simulink model "wrapper_ASW"  (R2024b)
settings: Solver=FixedStepDiscrete  StartTime=0.0  StopTime=10.0  FixedStep=0.001  MaxStep=0.001  RelTol=1e-3
libraries: simulink x2, CTRL x1, ESTS x1, INP x1, FUSI x1, OUT x1
settings Model: Creator=blatak  LastModifiedBy=blatak
settings ModelReferenceCC: EnableRefExpFcnMdlSchedulingChecks=on
settings RTWCC: GPUComputeCapability=3.5

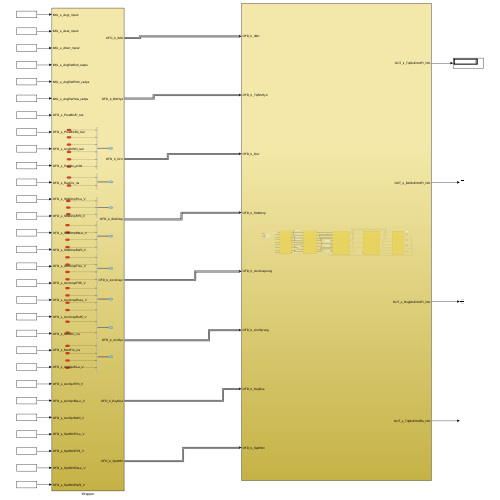
[thumbnail: Simulink's stored preview of the top-level diagram]
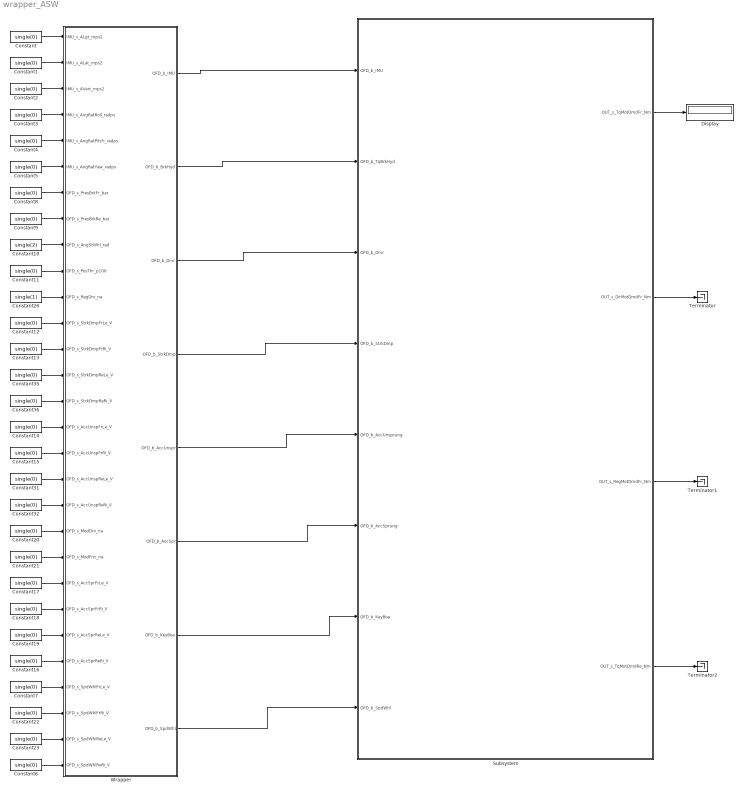
== system wrapper_ASW ==
  Constant{,1..9,11..23,31..32,35..36} (27 alike) : Constant  Value=single(0)
  Constant10 : Constant  Value=single(2)
  Constant26 : Constant  Value=single(1)
  Display : Display
  Subsystem : Subsystem
  Terminator : Terminator
  Terminator1 : Terminator
  Terminator2 : Terminator
  Wrapper : Subsystem
  wires:
  Wrapper/1(OFD_b_IMU) -> Subsystem/1(OFD_b_IMU)
  Wrapper/2(OFD_b_BrkHyd) -> Subsystem/2(OFD_b_TqBrkHyd)
  Wrapper/3(OFD_b_Drvr) -> Subsystem/3(OFD_b_Drvr)
  Wrapper/7(OFD_b_KeyBoa) -> Subsystem/7(OFD_b_KeyBoa)
  Constant/1 -> Wrapper/1(IMU_s_ALgt_mps2)
  Constant1/1 -> Wrapper/2(IMU_s_ALat_mps2)
  Constant2/1 -> Wrapper/3(IMU_s_AVert_mps2)
  Constant3/1 -> Wrapper/4(IMU_s_AngRatRoll_radps)
  Constant4/1 -> Wrapper/5(IMU_s_AngRatPitch_radps)
  Constant5/1 -> Wrapper/6(IMU_s_AngRatYaw_radps)
  Constant8/1 -> Wrapper/7(OFD_s_PresBrkFr_bar)
  Constant9/1 -> Wrapper/8(OFD_s_PresBrkRe_bar)
  Constant10/1 -> Wrapper/9(OFD_s_AngStWhl_rad)
  Constant11/1 -> Wrapper/10(OFD_s_PosThr_p100)
  Constant12/1 -> Wrapper/12(OFD_s_StrkDmpFrLe_V)
  Constant13/1 -> Wrapper/13(OFD_s_StrkDmpFrRi_V)
  Constant14/1 -> Wrapper/16(OFD_s_AccUnspFrLe_V)
  Constant15/1 -> Wrapper/17(OFD_s_AccUnspFrRi_V)
  Constant20/1 -> Wrapper/20(OFD_s_ModDrv_na)
  Constant21/1 -> Wrapper/21(OFD_s_ModFric_na)
  Constant26/1 -> Wrapper/11(OFD_s_RegDrv_na)
  Subsystem/1(OUT_s_TqMotDmdFr_Nm) -> Display/1
  Subsystem/2(OUT_s_DirMotDmdFr_Nm) -> Terminator/1
  Subsystem/3(OUT_s_RegMotDmdFr_Nm) -> Terminator1/1
  Subsystem/4(OUT_s_TqMotDmdRe_Nm) -> Terminator2/1
  Constant31/1 -> Wrapper/18(OFD_s_AccUnspReLe_V)
  Constant32/1 -> Wrapper/19(OFD_s_AccUnspReRi_V)
  Constant35/1 -> Wrapper/14(OFD_s_StrkDmpReLe_V)
  Constant36/1 -> Wrapper/15(OFD_s_StrkDmpReRi_V)
  Constant17/1 -> Wrapper/22(OFD_s_AccSprFrLe_V)
  Constant18/1 -> Wrapper/23(OFD_s_AccSprFrRi_V)
  Constant19/1 -> Wrapper/24(OFD_s_AccSprReLe_V)
  Constant16/1 -> Wrapper/25(OFD_s_AccSprReRi_V)
  Wrapper/6(OFD_b_AccSpr) -> Subsystem/6(OFD_b_AccSprung)
  Wrapper/5(OFD_b_AccUnspr) -> Subsystem/5(OFD_b_AccUnsprung)
  Wrapper/4(OFD_b_StrkDmp) -> Subsystem/4(OFD_b_StrkDmp)
  Constant7/1 -> Wrapper/26(OFD_s_SpdWhlFrLe_V)
  Constant22/1 -> Wrapper/27(OFD_s_SpdWhlFrRi_V)
  Constant23/1 -> Wrapper/28(OFD_s_SpdWhlReLe_V)
  Constant6/1 -> Wrapper/29(OFD_s_SpdWhlReRi_V)
  Wrapper/8(OFD_b_SpdWhl) -> Subsystem/8(OFD_b_SpdWhl)

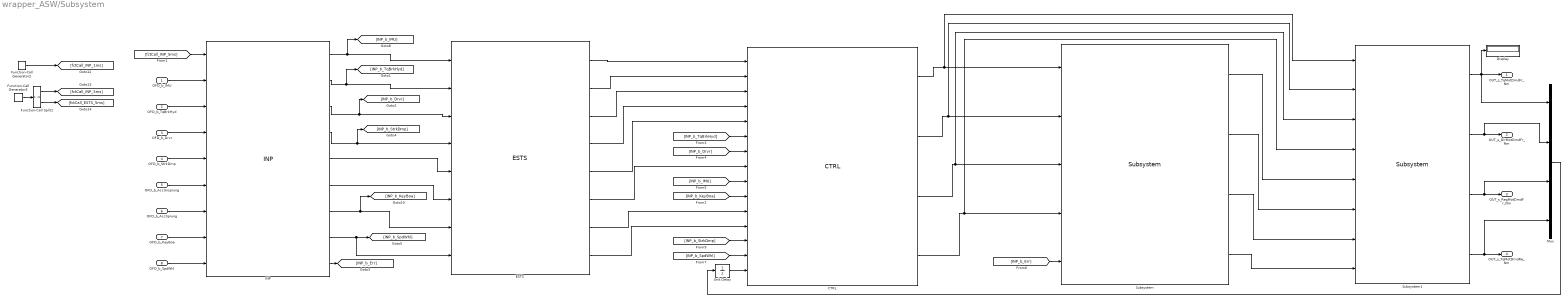
== system wrapper_ASW/Subsystem ==
  OFD_b_IMU : Inport
  OFD_b_TqBrkHyd : Inport  Port=2
  OFD_b_Drvr : Inport  Port=3
  OFD_b_StrkDmp : Inport  Port=4
  OFD_b_AccUnsprung : Inport  Port=5
  OFD_b_AccSprung : Inport  Port=6
  OFD_b_KeyBoa : Inport  Port=7
  OFD_b_SpdWhl : Inport  Port=8
  CTRL : CTRL/CTRL  SystemSampleTime=-1  VariantActivationTime=update diagram  AllowFlexibleInterface=on  Latency=0  AutoFrameSizeCalculation=off
  Display : Display
  ESTS : ESTS/ESTS  SystemSampleTime=-1  VariantActivationTime=update diagram  AllowFlexibleInterface=on  Latency=0  AutoFrameSizeCalculation=off
  Function-Call Generator2 : simulink/Ports & Subsystems/Function-Call Generator  sample_time=1  numberOfIterations=1  DisallowWideOutput=off
  Function-Call Generator3 : simulink/Ports & Subsystems/Function-Call Generator  sample_time=0.005  numberOfIterations=1  DisallowWideOutput=off
  Function-Call Split1 : FunctionCallSplit  IconShape=distinctive  NumOutputPorts=2  OutputPortLayout=default
  INP : INP/INP  SystemSampleTime=-1  VariantActivationTime=update diagram  AllowFlexibleInterface=on  Latency=0  AutoFrameSizeCalculation=off
      link override Function-Call Subsystem1/Bus Selector2: OutputSignals=OFD_s_AngStWhl_rad,OFD_s_PosThr_p100,OFD_s_RegDrv_na
  Mux : Mux
  Subsystem : FUSI/Subsystem  SystemSampleTime=-1  VariantActivationTime=update diagram  AllowFlexibleInterface=on  Latency=0  AutoFrameSizeCalculation=off
  Subsystem1 : OUT/Subsystem  SystemSampleTime=-1  VariantActivationTime=update diagram  AllowFlexibleInterface=on  Latency=0  AutoFrameSizeCalculation=off
  Unit Delay : UnitDelay  SampleTime=-1  HasFrameUpgradeWarning=on
  OUT_s_TqMotDmdFr_Nm : Outport
  OUT_s_DirMotDmdFr_Nm : Outport  Port=2
  OUT_s_RegMotDmdFr_Nm : Outport  Port=3
  OUT_s_TqMotDmdRe_Nm : Outport  Port=4
  wires:
  OFD_b_IMU/1 -> INP/2
  [fctCall_INP_5ms] -> INP/1
  OFD_b_Drvr/1 -> INP/4
  INP/3 -> [INP_b_Drvr], ESTS/3
  Function-Call Generator2/1 -> [fctCall_INP_1ms]
  Function-Call Generator3/1 -> Function-Call Split1/1
  INP/1 -> ESTS/1, [INP_b_IMU]
  Function-Call Split1/1 -> [fctCall_INP_5ms]
  Function-Call Split1/2 -> [fctCall_ESTS_5ms]
  ESTS/7 -> CTRL/11
  [INP_b_KeyBoa] -> CTRL/10
  [INP_b_Drvr] -> CTRL/7
  [INP_b_TqBrkHyd] -> CTRL/6
  ESTS/6 -> CTRL/8
  [INP_b_IMU] -> CTRL/9
  CTRL/1 -> Subsystem1/1, Subsystem/1
  CTRL/2 -> Subsystem1/2, Subsystem/2
  CTRL/3 -> Subsystem1/3, Subsystem/3
  CTRL/4 -> Subsystem1/4, Subsystem/4
  Subsystem1/1 -> Display/1, Mux/1, OUT_s_TqMotDmdFr_Nm/1
  Subsystem1/2 -> Mux/2, OUT_s_DirMotDmdFr_Nm/1
  Subsystem1/3 -> Mux/3, OUT_s_RegMotDmdFr_Nm/1
  Subsystem1/4 -> Mux/4, OUT_s_TqMotDmdRe_Nm/1
  [INP_b_StrkDmp] -> CTRL/13
  OFD_b_TqBrkHyd/1 -> INP/3
  OFD_b_StrkDmp/1 -> INP/5
  OFD_b_AccUnsprung/1 -> INP/6
  OFD_b_AccSprung/1 -> INP/7
  OFD_b_KeyBoa/1 -> INP/8
  INP/2 -> ESTS/2, [INP_b_TqBrkHyd]
  INP/4 -> [INP_b_StrkDmp], ESTS/4
  INP/5 -> ESTS/5
  INP/6 -> ESTS/6
  INP/7 -> ESTS/7, [INP_b_KeyBoa]
  ESTS/1 -> CTRL/1
  ESTS/2 -> CTRL/2
  ESTS/3 -> CTRL/3
  ESTS/4 -> CTRL/4
  ESTS/5 -> CTRL/5
  ESTS/8 -> CTRL/12
  [INP_b_Err] -> Subsystem/5
  Subsystem/1 -> Subsystem1/5
  Subsystem/2 -> Subsystem1/6
  Subsystem/3 -> Subsystem1/7
  Subsystem/4 -> Subsystem1/8
  OFD_b_SpdWhl/1 -> INP/9
  INP/8 -> [INP_b_SpdWhl], ESTS/8
  INP/9 -> [INP_b_Err]
  [INP_b_SpdWhl] -> CTRL/14
  Mux/1 -> Unit Delay/1
  Unit Delay/1 -> CTRL/15

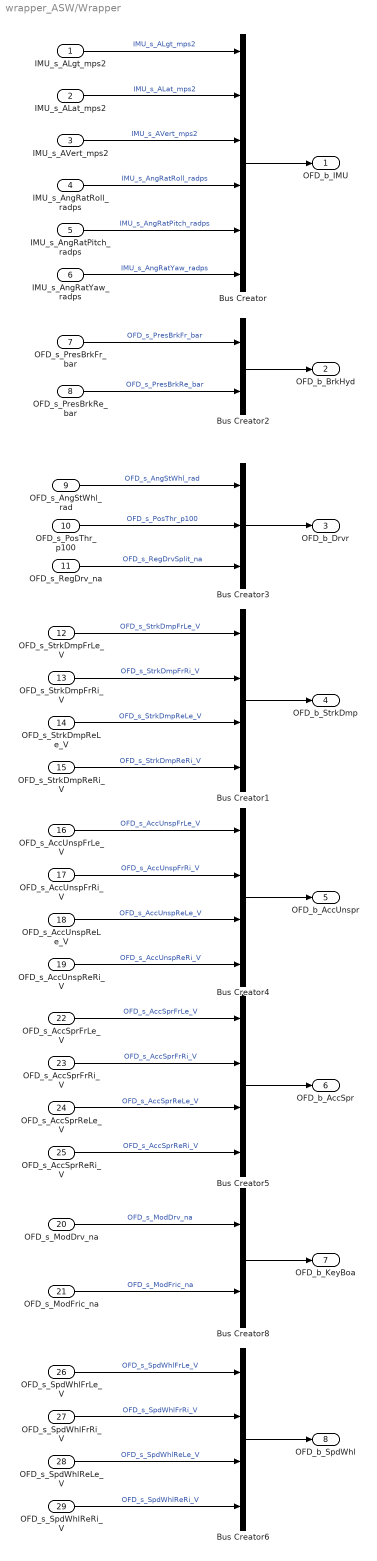
== system wrapper_ASW/Wrapper ==
  IMU_s_ALgt_mps2 : Inport
  IMU_s_ALat_mps2 : Inport  Port=2
  IMU_s_AVert_mps2 : Inport  Port=3
  IMU_s_AngRatRoll_radps : Inport  Port=4
  IMU_s_AngRatPitch_radps : Inport  Port=5
  IMU_s_AngRatYaw_radps : Inport  Port=6
  OFD_s_PresBrkFr_bar : Inport  Port=7
  OFD_s_PresBrkRe_bar : Inport  Port=8
  OFD_s_AngStWhl_rad : Inport  Port=9
  OFD_s_PosThr_p100 : Inport  Port=10
  OFD_s_RegDrv_na : Inport  Port=11
  OFD_s_StrkDmpFrLe_V : Inport  Port=12
  OFD_s_StrkDmpFrRi_V : Inport  Port=13
  OFD_s_StrkDmpReLe_V : Inport  Port=14
  OFD_s_StrkDmpReRi_V : Inport  Port=15
  OFD_s_AccUnspFrLe_V : Inport  Port=16
  OFD_s_AccUnspFrRi_V : Inport  Port=17
  OFD_s_AccUnspReLe_V : Inport  Port=18
  OFD_s_AccUnspReRi_V : Inport  Port=19
  OFD_s_ModDrv_na : Inport  Port=20
  OFD_s_ModFric_na : Inport  Port=21
  OFD_s_AccSprFrLe_V : Inport  Port=22
  OFD_s_AccSprFrRi_V : Inport  Port=23
  OFD_s_AccSprReLe_V : Inport  Port=24
  OFD_s_AccSprReRi_V : Inport  Port=25
  OFD_s_SpdWhlFrLe_V : Inport  Port=26
  OFD_s_SpdWhlFrRi_V : Inport  Port=27
  OFD_s_SpdWhlReLe_V : Inport  Port=28
  OFD_s_SpdWhlReRi_V : Inport  Port=29
  Bus Creator : BusCreator  Inputs=6  OutDataTypeStr=Bus: OFD_b_IMU
      settings: InheritFromInputs=off
  Bus Creator1 : BusCreator  Inputs=4  OutDataTypeStr=Bus: OFD_b_StrkDmp
      settings: InheritFromInputs=off
  Bus Creator2 : BusCreator  Inputs=2  OutDataTypeStr=Bus: OFD_b_TqBrkHyd
      settings: InheritFromInputs=off
  Bus Creator3 : BusCreator  Inputs=3  OutDataTypeStr=Bus: OFD_b_Drvr
      settings: InheritFromInputs=off
  Bus Creator4 : BusCreator  Inputs=4  OutDataTypeStr=Bus: OFD_b_AccUnsp
      settings: InheritFromInputs=off
  Bus Creator5 : BusCreator  Inputs=4  OutDataTypeStr=Bus: OFD_b_AccSpr
      settings: InheritFromInputs=off
  Bus Creator6 : BusCreator  Inputs=4  OutDataTypeStr=Bus: OFD_b_SpdWhl
      settings: InheritFromInputs=off
  Bus Creator8 : BusCreator  Inputs=2  OutDataTypeStr=Bus: OFD_b_KeyBoa
      settings: InheritFromInputs=off
  OFD_b_IMU : Outport
  OFD_b_BrkHyd : Outport  Port=2
  OFD_b_Drvr : Outport  Port=3
  OFD_b_StrkDmp : Outport  Port=4
  OFD_b_AccUnspr : Outport  Port=5
  OFD_b_AccSpr : Outport  Port=6
  OFD_b_KeyBoa : Outport  Port=7
  OFD_b_SpdWhl : Outport  Port=8
  wires:
  IMU_s_ALgt_mps2/1 -> Bus Creator/1  "IMU_s_ALgt_mps2"
  IMU_s_AngRatYaw_radps/1 -> Bus Creator/6  "IMU_s_AngRatYaw_radps"
  IMU_s_AngRatPitch_radps/1 -> Bus Creator/5  "IMU_s_AngRatPitch_radps"
  IMU_s_AngRatRoll_radps/1 -> Bus Creator/4  "IMU_s_AngRatRoll_radps"
  IMU_s_AVert_mps2/1 -> Bus Creator/3  "IMU_s_AVert_mps2"
  IMU_s_ALat_mps2/1 -> Bus Creator/2  "IMU_s_ALat_mps2"
  Bus Creator/1 -> OFD_b_IMU/1
  OFD_s_PresBrkFr_bar/1 -> Bus Creator2/1  "OFD_s_PresBrkFr_bar"
  OFD_s_PresBrkRe_bar/1 -> Bus Creator2/2  "OFD_s_PresBrkRe_bar"
  Bus Creator2/1 -> OFD_b_BrkHyd/1
  OFD_s_AngStWhl_rad/1 -> Bus Creator3/1  "OFD_s_AngStWhl_rad"
  OFD_s_PosThr_p100/1 -> Bus Creator3/2  "OFD_s_PosThr_p100"
  OFD_s_AccUnspFrLe_V/1 -> Bus Creator4/1  "OFD_s_AccUnspFrLe_V"
  OFD_s_AccUnspFrRi_V/1 -> Bus Creator4/2  "OFD_s_AccUnspFrRi_V"
  OFD_s_StrkDmpFrRi_V/1 -> Bus Creator1/2  "OFD_s_StrkDmpFrRi_V"
  OFD_s_StrkDmpFrLe_V/1 -> Bus Creator1/1  "OFD_s_StrkDmpFrLe_V"
  Bus Creator3/1 -> OFD_b_Drvr/1
  Bus Creator4/1 -> OFD_b_AccUnspr/1
  OFD_s_ModFric_na/1 -> Bus Creator8/2  "OFD_s_ModFric_na"
  OFD_s_ModDrv_na/1 -> Bus Creator8/1  "OFD_s_ModDrv_na"
  Bus Creator8/1 -> OFD_b_KeyBoa/1
  OFD_s_RegDrv_na/1 -> Bus Creator3/3  "OFD_s_RegDrvSplit_na"
  OFD_s_AccUnspReLe_V/1 -> Bus Creator4/3  "OFD_s_AccUnspReLe_V"
  OFD_s_AccUnspReRi_V/1 -> Bus Creator4/4  "OFD_s_AccUnspReRi_V"
  OFD_s_AccSprReRi_V/1 -> Bus Creator5/4  "OFD_s_AccSprReRi_V"
  OFD_s_AccSprFrRi_V/1 -> Bus Creator5/2  "OFD_s_AccSprFrRi_V"
  OFD_s_AccSprReLe_V/1 -> Bus Creator5/3  "OFD_s_AccSprReLe_V"
  OFD_s_AccSprFrLe_V/1 -> Bus Creator5/1  "OFD_s_AccSprFrLe_V"
  OFD_s_StrkDmpReLe_V/1 -> Bus Creator1/3  "OFD_s_StrkDmpReLe_V"
  OFD_s_StrkDmpReRi_V/1 -> Bus Creator1/4  "OFD_s_StrkDmpReRi_V"
  Bus Creator1/1 -> OFD_b_StrkDmp/1
  Bus Creator5/1 -> OFD_b_AccSpr/1
  OFD_s_SpdWhlFrLe_V/1 -> Bus Creator6/1  "OFD_s_SpdWhlFrLe_V"
  OFD_s_SpdWhlFrRi_V/1 -> Bus Creator6/2  "OFD_s_SpdWhlFrRi_V"
  Bus Creator6/1 -> OFD_b_SpdWhl/1
  OFD_s_SpdWhlReLe_V/1 -> Bus Creator6/3  "OFD_s_SpdWhlReLe_V"
  OFD_s_SpdWhlReRi_V/1 -> Bus Creator6/4  "OFD_s_SpdWhlReRi_V"
